simulink model "connection5_second"  (R2017b)
settings: Solver=VariableStepAuto  StartTime=0.0  StopTime=50.0  RelTol=1e-3
values from neighbouring files (symbols this model uses):
  A5 = [-2,0,0,0,0,0,0,0,1,0 ... (first row only)    [param.m]
  D2_5 = [(d2(1,1)-d2(5,1))+d2(1,1) ... (first row only)    [param.m]
  K1 = 1    [param.m]
  start = [0;1.5;0;-1.5;-3;3;-3;0;-3;-3]    [param.m]
settings Model: Creator=yunfei  LastModifiedBy=yunfei

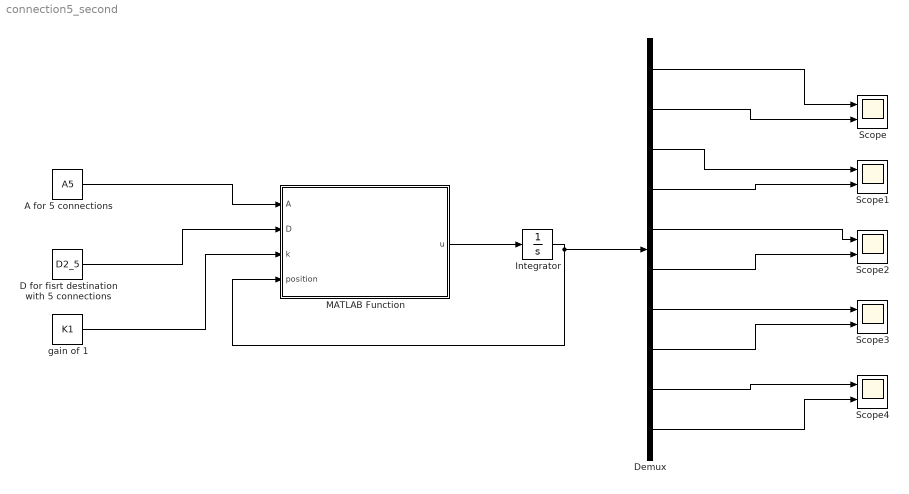
== system connection5_second ==
  A for 5 connections : Constant  Value=A5
  "D for fisrt destination with 5 connections " : Constant  Value=D2_5
  Demux : Demux  Outputs=10
  Integrator : Integrator  InitialCondition=start
  MATLAB Function : MATLAB Function  TreatAsAtomicUnit=on
  Scope{,1..4} (5 alike) : Scope  NumInputPorts=2
  gain of 1 : Constant  Value=K1
  wires:
  Demux/6 -> Scope2/2
  Demux/10 -> Scope4/2
  Demux/5 -> Scope2/1
  Demux/8 -> Scope3/2
  Integrator/1 -> MATLAB Function/4(position), Demux/1
  Demux/4 -> Scope1/2
  MATLAB Function/1(u) -> Integrator/1
  Demux/7 -> Scope3/1
  Demux/9 -> Scope4/1
  "D for fisrt destination with 5 connections "/1 -> MATLAB Function/2(D)
  Demux/1 -> Scope/1
  A for 5 connections/1 -> MATLAB Function/1(A)
  Demux/2 -> Scope/2
  Demux/3 -> Scope1/1
  gain of 1/1 -> MATLAB Function/3(k)

== matlab function connection5_second/MATLAB Function ==
  data: A input; u output; D input; k input; position input
function u = fcn(A, D, k, position)
    u = k.*A * position + D;
end
